simulink model "simulation_poly_new"  (R2015b)
settings: Solver=ode45  StartTime=0.0  StopTime=5.5  RelTol=1e-3
settings Model: Creator=Παναγιώτης Κυριάκης  LastModifiedBy=Panagiotis Kyriakis
settings DataIOCC: SaveFormat=Array
settings HardwareCC: ProdBitPerPointer=32  ProdLargestAtomicFloat=None  ProdIntDivRoundTo=Undefined  ProdEndianess=Unspecified  ProdWordSize=32  ProdHWDeviceType=32-bit Generic
settings GRTTargetCC: GeneratePreprocessorConditionals=Disable all
settings ConfigComp: CovModelRefEnable=Off

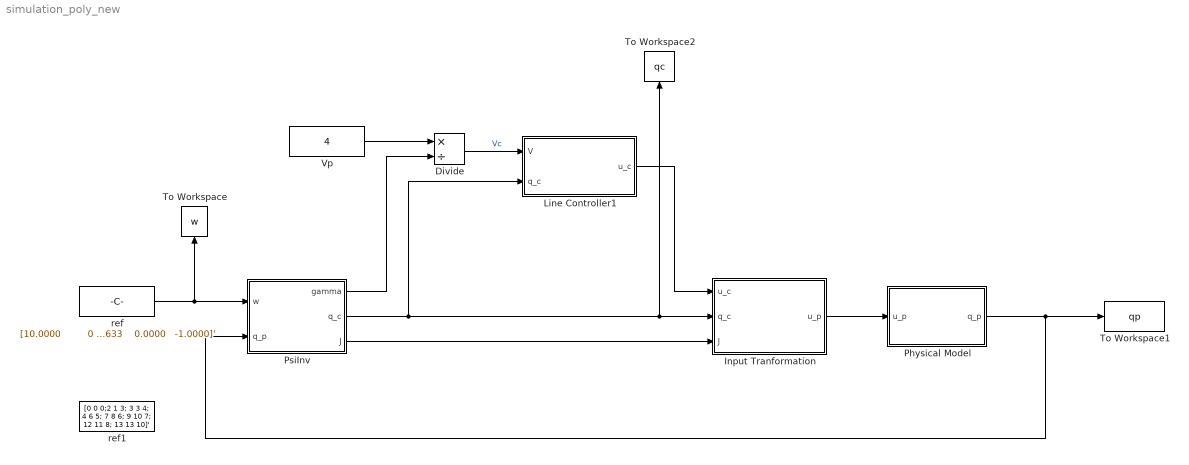
== system simulation_poly_new ==
  Divide : Product  Inputs=*/
  "Input Tranformation " : MATLAB Function  TreatAsAtomicUnit=on
  Line Controller1 : MATLAB Function  TreatAsAtomicUnit=on
  Physical Model : Subsystem
  PsiInv : MATLAB Function  TreatAsAtomicUnit=on
  To Workspace : ToWorkspace  VariableName=w  SaveFormat=Timeseries  SampleTime=-1
  To Workspace1 : ToWorkspace  VariableName=qp  SaveFormat=Timeseries  SampleTime=-1
  To Workspace2 : ToWorkspace  VariableName=qc  SaveFormat=Timeseries  SampleTime=-1
  Vp : Constant  Value=4
  ref : Constant  Value=|  VectorParams1D=off  LockScale=on
      | [10.0000         0    1.0000;
      |    10.6964    0.6235    0.7818;
      |    11.4412    0.9749    0.2225
      | ;   12.2380    0.9010   -0.4339
      |   ; 13.0902    0.4339   -0.9010
      | ;   14.0018   -0.2225   -0.9749;
      |    14.9768   -0.7818   -0.6235
      | ;   16.0198   -1.0000   -0.0000
      |   ; 17.1354   -0.7818    0.6235
      | ;   18.3286   -0.2225    0.9749
      |  ;  19.6050    0.4339    0.9010
      |  ;  20.9702    0.9010    0.4339
      |  ;  22.4305    0.9749   -0.2225
      | ;   23.9925    0.6235   -0.7818
      | ;   25.6633    0.0000   -1.0000]'
  ref1 : Constant  Value=[0 0 0;2 1 3; 3 3 4; 4 6 5; 7 8 6; 9 10 7; 12 11 8; 13 13 10]'  VectorParams1D=off  LockScale=on
  wires:
  PsiInv/2(q_c) -> "Input Tranformation "/2(q_c), To Workspace2/1, Line Controller1/2(q_c)
  "Input Tranformation "/1(u_p) -> Physical Model/1(u_p)
  Physical Model/1(q_p) -> PsiInv/2(q_p), To Workspace1/1
  PsiInv/3(J) -> "Input Tranformation "/3(J)
  Line Controller1/1(u_c) -> "Input Tranformation "/1(u_c)
  ref/1 -> To Workspace/1, PsiInv/1(w)
  PsiInv/1(gamma) -> Divide/2
  Vp/1 -> Divide/1
  Divide/1 -> Line Controller1/1(V)  "Vc"

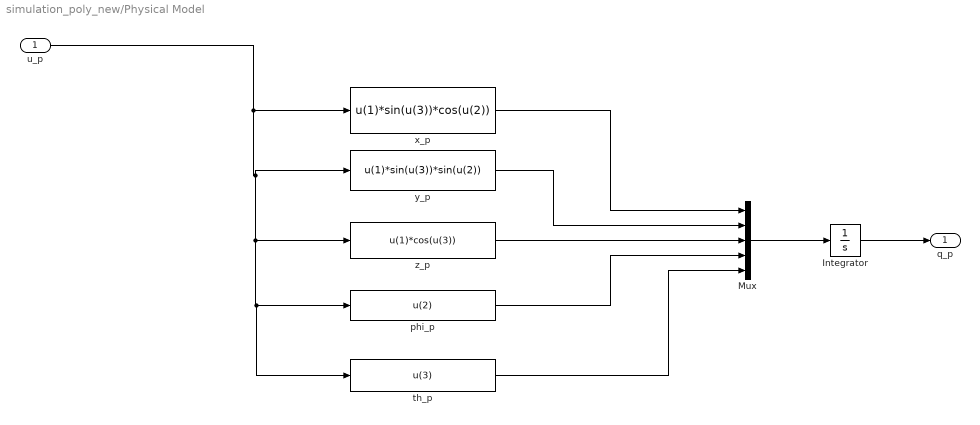
== system simulation_poly_new/Physical Model ==
  u_p : Inport
  Integrator : Integrator  InitialCondition=[9 -0.8 -0.5 pi/2 pi/9]  UpperSaturationLimit=1000  LowerSaturationLimit=-1000
  Mux : Mux  Inputs=5
  phi_p : Fcn  Expr=u(2)
  th_p : Fcn  Expr=u(3)
  "x_p " : Fcn  Expr=u(1)*sin(u(3))*cos(u(2))
  y_p : Fcn  Expr=u(1)*sin(u(3))*sin(u(2))
  z_p : Fcn  Expr=u(1)*cos(u(3))
  q_p : Outport
  wires:
  y_p/1 -> Mux/2
  z_p/1 -> Mux/3
  th_p/1 -> Mux/5
  Integrator/1 -> q_p/1
  "x_p "/1 -> Mux/1
  phi_p/1 -> Mux/4
  Mux/1 -> Integrator/1
  u_p/1 -> th_p/1, phi_p/1, z_p/1, y_p/1, "x_p "/1

== matlab function simulation_poly_new/PsiInv ==
  data: gamma output; w input; q_p input; q_c output; J output
function [gamma,q_c, J]   = PsiInv(w,q_p)
    
%     w = zeros(3,10);
%     w = [0 0 0;2 1 3; 3 3 4; 4 6 5; 7 8 6; 9 10 7; 12 11 8; 13 13 10]';
    persistent a Ss  
    Ss=sum(diff(w,1,2).^2);
    a=[0 cumsum(Ss)/sum(Ss)];
% a = [0 0.1658 0.2744 0.4213 0.5871 0.7201 0.8671 1];
    
    rp = q_p(1:3,1);
    n = max(size(w));
    v = zeros(3,n-1);
    S = 0;
    
    % Compute v and S
    for k=1:n-1
        v(:,k)=(w(:,k+1)-w(:,k))/norm(w(:,k+1)-w(:,k));
        S = S + sqrt((w(:,k)-w(:,k+1))'*(w(:,k)-w(:,k+1)));
    end
    
    % Find active edge
    K = 0;
    uy = [0 1 0]';
    uz = [0 0 1]';
    N = cross(uy,uz);
    for k=1:n-1
        d1 = (N')*(rp-w(:,k));
        d2 = (N')*(rp-w(:,k+1));
        if(d1*d2<=0)
            K=k;
            break;
        end              
    end
    
    if (K == 0)
        wtmp = w(:,n) + 100000*v(:,n-1);
        d1 = (N')*(rp-w(:,n));
        d2 = (N')*(rp-wtmp);
        if(d1*d2<0)
            K=n;
        end     
    end
    
    % Find Jacobian
    J = zeros(3,3);
    J(:,2) = S*uy;
    J(:,3) = S*uz;
    
    % Find canoncical r
    if (K == 0)
        J(:,1) = S*v(:,1);
        r_c = J\(rp-w(:,1)+S*a(1)*v(:,1));
    elseif (K == n)
        J(:,1) = S*v(:,n-1);
        r_c = J\(rp-w(:,K)+S*a(K)*v(:,n-1));
    else
        J(:,1) = S*v(:,K);
        r_c = J\(rp-w(:,K)+S*a(K)*v(:,K));
    end
    
    % Get physical angles and their unit vector
    th_p = q_p(5);
    phi_p = q_p(4);
    cp = [sin(th_p)*cos(phi_p);
          sin(th_p)*sin(phi_p);
          cos(th_p)];
    
    % Find canonical phi, th   
    cc = J\cp/norm(J\cp);    
    phi_c = atan2(cc(2),cc(1));
    th_c = acos(cc(3));   
    
    % calculate gamma);
    gamma = sqrt(cc'*(J'*J)*cc);
    % Canonical space-state vector
    q_c =[r_c;phi_c;th_c];   
end

== matlab function simulation_poly_new/Input Tranformation  ==
  data: u_c input; q_c input; J input; u_p output
function u_p = M(u_c,q_c,J)
    
    % Initialization
    C = zeros(2,3);
    D = eye(2);
    M = eye(3);
    Jd = zeros(3,3);
    
    % Construct needed elements of Cartesian tensor
    e12=[1 0 0]'*[0 1 0];
    e21=[0 1 0]'*[1 0 0];
    e33=[0 0 1]'*[0 0 1];
    
    % Get canonical angles
    th_c = q_c(5);
    phi_c = q_c(4);    
    
    % Construct the vector cc and its derivatives
    cc = [sin(th_c)*cos(phi_c);
          sin(th_c)*sin(phi_c);
          cos(th_c)];
    cc_phi_c = [-sin(th_c)*sin(phi_c);
                 sin(th_c)*cos(phi_c);
                 0];
    cc_th_c = [cos(th_c)*cos(phi_c);
               cos(th_c)*sin(phi_c);
               -sin(th_c)];
    
    % Find the length ratio
    gamma = sqrt(cc'*(J'*J)*cc);

    % Find the coefficients appearing in C,D
    Aphi = (cc')*(J')*(e12-e21)/(gamma^2-cc'*J'*e33*J*cc);
    Ath = -gamma*[0 0 1]/sqrt(gamma^2-cc'*J'*e33*J*cc);

    % Find C
    C(1,1) = Aphi*Jd*cc;
    C(2,1) = Ath*(2*(gamma^2)*Jd-cc'*(Jd'*J+J'*Jd)*cc*J)*cc/(2*gamma^3);
 
    % Find D
    D(1,1) = Aphi*J*cc_phi_c;
    D(1,2) = Aphi*J*cc_th_c;
    D(2,1) = Ath*J*(cc_phi_c*cc'-cc*cc_phi_c')*J'*J*cc/gamma^3;
    D(2,2) = Ath*J*(cc_th_c*cc'-cc*cc_th_c')*J'*J*cc/gamma^3;
    % Find M

    M(1,1) = gamma;
    M(2:3,1) = C*cc;
    M(2:3,2:3) = D;

    % Transform the control
    u_p = M*u_c;
    phi_dot_max = 20;
    th_dot_max=2.2;
    if(u_p(2)>phi_dot_max) 
        u_p(2)=phi_dot_max;
    end
    if(u_p(2)<-phi_dot_max) 
        u_p(2)=-phi_dot_max;
    end
    if(u_p(3)>th_dot_max) 
        u_p(3)=th_dot_max;
    end
    if(u_p(3)<-th_dot_max) 
        u_p(3)=-th_dot_max;
    end

    
 end

== matlab function simulation_poly_new/Line Controller1 ==
  data: V input; q_c input; u_c output
function u_c = LineCon(V,q_c)

    K2 = -0.04*[1;0;0]; 
    r_c = [0; q_c(2); q_c(3)];
        
    v = -5*r_c - K2;
    v=V*v/norm(v);
    
    u_c = [ V; 
            atan2(v(2),v(1));
            acos(v(3)/V)];  
        
end
